simulink model "Location_plot"  (R2023a)
settings: Solver=FixedStepDiscrete  StartTime=0.0  StopTime=inf  RelTol=1e-3
libraries: androidcommunicationlib x2, visionsources x1, androidaudiovideolib x1
settings Model: Creator=Aryan  LastModifiedBy=Aryan
settings OptimizationCC: EnhancedBackFolding=on  PassReuseOutputArgsAs=Individual arguments  ZeroExternalMemoryAtStartup=off  ZeroInternalMemoryAtStartup=off  MaxStackSize=64  OptimizeBlockOrder=speed  DifferentSizesBufferReuse=on  OptimizationCustomize=off  EfficientTunableParamExpr=on
settings DebuggingCC: ParameterTunabilityLossMsg=error
settings HardwareCC: ProdBitPerPointer=32  ProdBitPerSizeT=32  ProdBitPerPtrDiffT=32  ProdLargestAtomicInteger=Long  ProdLargestAtomicFloat=Double  ProdWordSize=32  ProdHWDeviceType=ARM Compatible->ARM Cortex
settings SFSimCC: MATLABDynamicMemAlloc=off
settings RTWCC: Description=Embedded Coder  SystemTargetFile=ert.tlc  HardwareBoard=Android Device  TLCOptions="-aInlineSetEventsForThisBaseRateFcn=TLC_FALSE -aSuppressMultiTaskScheduler=TLC_FALSE  -aRateBasedStepFcn=0"  TemplateMakefile=ert_default_tmf  RTWVerbose=off  Toolchain=Android SDK/NDK Tools
settings CodeAppCC: ForceParamTrailComments=on  IgnoreCustomStorageClasses=off  OperatorAnnotations=on  SimulinkDataObjDesc=on  SFDataObjDesc=on  InsertBlockDesc=on

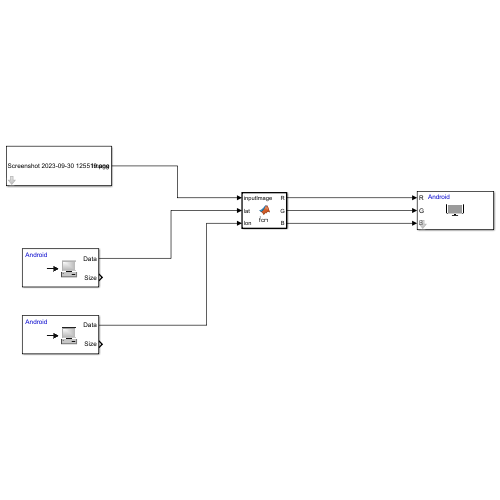
[thumbnail: Simulink's stored preview of the top-level diagram]
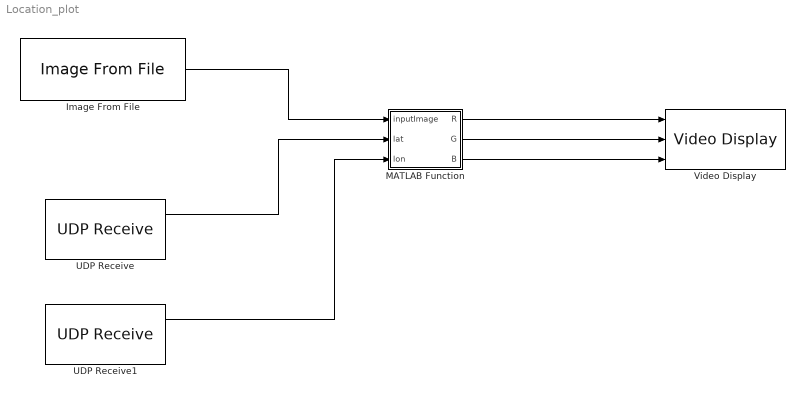
== system Location_plot ==
  Image From File : visionsources/Image From File  Tag=vipblks_nd  FileName=C:\Users\aryan\OneDrive\Pictures\Screenshots\Screenshot 2023-09-30 125519.png  Ts=inf  imagePorts=One multidimensional signal  OutPortLabels=R|G|B  ImageDataType=Inherit from input image  sdImageDataType=uint(8)  Signed=on  WordLength=16  FractionLengthMode=User-defined  FractionLength=15
  MATLAB Function : MATLAB Function  TreatAsAtomicUnit=on
  UDP Receive : androidcommunicationlib/UDP Receive  localURL='0.0.0.0'  localPort=25000  remoteURL='0.0.0.0'  remotePort=-1  recvBufferSize=8192  signalDatatype=uint8  dims=1  isVarSize=off  showBlockingTime=off  blockingTime=0  sampletime=0.01  blockPlatform=Android
  UDP Receive1 : androidcommunicationlib/UDP Receive  localURL='0.0.0.0'  localPort=25001  remoteURL='0.0.0.0'  remotePort=-1  recvBufferSize=8192  signalDatatype=uint8  dims=1  isVarSize=off  showBlockingTime=off  blockingTime=0  sampletime=0.01  blockPlatform=Android
  Video Display : androidaudiovideolib/Video Display  BlockPlatform=Android
  wires:
  Image From File/1 -> MATLAB Function/1(inputImage)
  MATLAB Function/1(R) -> Video Display/1
  MATLAB Function/2(G) -> Video Display/2
  MATLAB Function/3(B) -> Video Display/3
  UDP Receive/1 -> MATLAB Function/2(lat)
  UDP Receive1/1 -> MATLAB Function/3(lon)

== matlab function Location_plot/MATLAB Function ==
  data: inputImage input; R output; lat input; lon input; G output; B output
function [R,G,B] = fcn(inputImage,lat,lon)

x=floor((lat-23.20856)*(507/(23.21318-23.20856)));
y=469-floor((lon-72.68223)*(469/(72.68759-72.68223)));


% Add a red marker (a red dot) at the specified coordinates
processedImage = inputImage; % Create a copy of the input image
processedImage(y-10:y+10, x-10:x+10, 1) = 255; % Set the red channel to 255 at the marker location
processedImage(y-10:y+10, x-10:x+10, 2:3) = 0; % Set the green and blue channels to 0 at the marker location
processedImage=fliplr(processedImage);
imshow(processedImage);
R=processedImage(:,:,1);
G=processedImage(:,:,2);
B=processedImage(:,:,3);
